simulink model "systemIndentificationLinearR2019a"  (R2019a)
settings: Solver=FixedStepAuto  StartTime=0.0  StopTime=20  RelTol=1e-3  EnableMultiTasking=on
undefined symbols (not defined in the file): sigbuilder_block
libraries: arduinolib x7, simulink x1
settings Model: SimulationMode=external  ExtModeTrigDuration=2  Creator=Win7  LastModifiedBy=manh
settings DataIOCC: SaveFormat=Array  SaveOutput=off  SaveTime=off  ReturnWorkspaceOutputs=off
settings OptimizationCC: PassReuseOutputArgsAs=Individual arguments  MaxStackSize=64
settings DebuggingCC: ParameterTunabilityLossMsg=error  ArithmeticOperatorsInVariantConditions=warning
settings HardwareCC: ProdBitPerInt=16  ProdBitPerPointer=16  ProdBitPerSizeT=16  ProdBitPerPtrDiffT=16  ProdLargestAtomicFloat=None  ProdWordSize=8  ProdHWDeviceType=Atmel->AVR
settings SFSimCC: SimUseLocalCustomCode=off  MATLABDynamicMemAlloc=off
settings RTWCC: SystemTargetFile=ert.tlc  HardwareBoard=Arduino Mega 2560  TLCOptions=-aInlineSetEventsForThisBaseRateFcn=TLC_FALSE -aSuppressMultiTaskScheduler=TLC_FALSE -aRateBasedStepFcn=1  TemplateMakefile=ert_default_tmf  GenerateReport=on  RTWUseLocalCustomCode=off  Toolchain=Arduino AVR  BuildConfiguration=Faster Runs  IncludeHyperlinkInReport=on  LaunchReport=on  GenerateTraceInfo=on  GenerateTraceReport=on  GenerateTraceReportSl=on  GenerateTraceReportSf=on  GenerateTraceReportEml=on
settings CodeAppCC: ForceParamTrailComments=on  IgnoreCustomStorageClasses=off  OperatorAnnotations=on  SimulinkDataObjDesc=on  SFDataObjDesc=on  InsertBlockDesc=on
settings ERTTargetCC: SupportContinuousTime=on  SupportVariableSizeSignals=on

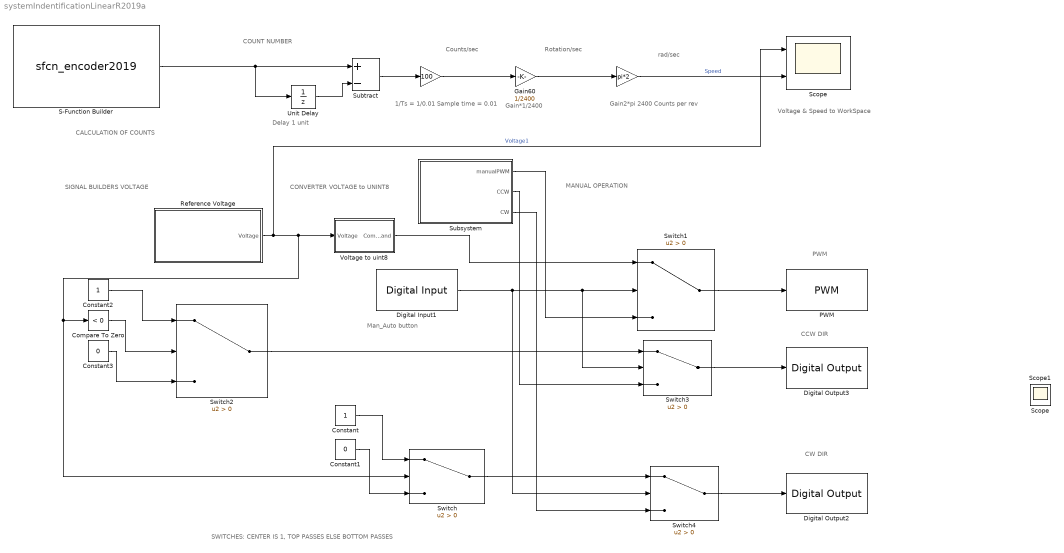
== system systemIndentificationLinearR2019a ==
  note: SIGNAL BUILDERS
      | VOLTAGE
  note: CALCULATION OF COUNTS
  note: SWITCHES: CENTER IS 1, TOP PASSES ELSE BOTTOM PASSES
  note: CONVERTER
      | VOLTAGE to UNINT8
  note: MANUAL OPERATION
  note: Voltage & Speed
      | to WorkSpace
  note: Gain2*pi
      | 2400 Counts per rev
  note: 1/Ts = 1/0.01
      | Sample time = 0.01
  note: Counts/sec
  note: Delay 1 unit
  note: CW DIR
  note: CCW DIR
  note: PWM
  note: Man_Auto button
  note: Rotation/sec
  note: rad/sec
  note: Gain*1/2400
  note: COUNT NUMBER
  " " : Gain  Gain=100  OutDataTypeStr=double
  " " : Gain  Gain=pi*2  OutDataTypeStr=double
  Compare To Zero : simulink/Logic and Bit Operations/Compare To Zero  relop=<  OutDataTypeStr=boolean
  Constant : Constant
  Constant1 : Constant  Value=0
  Constant2 : Constant
  Constant3 : Constant  Value=0
  Digital Input1 : arduinolib/Digital Input  pinNumber=28  sampleTime=0.01  blockPlatform=arduino
      settings: SourceProductName=Simulink Support Package for Arduino Hardware
  Digital Output2 : arduinolib/Digital Output  pinNumber=36  blockPlatform=arduino
  Digital Output3 : arduinolib/Digital Output  pinNumber=38  blockPlatform=arduino
  Gain60 : Gain  Gain=1/2400  OutDataTypeStr=double
  PWM : arduinolib/PWM  pinNumber=7  EnableInputFrequency=off  InitialFrequency=2000  InitialDutyCycle=0  NotificationType=None  blockPlatform=arduino
  Reference Voltage : Subsystem  Tag=STV Subsys  LoadFcn=sigbuilder_block('load');  StartFcn=sigbuilder_block('start');  StopFcn=sigbuilder_block('stop');  ClipboardFcn=sigbuilder_block('clipboard');  mask(Sigbuilder block){tuvar=[0:10]}
      mask help: Sigbuilder GUI
      mask init:
      | if ~strcmp(get_param(bdroot(gcbh),'SimulationStatus'),'stopped') tuvar = sigbuilder_block('maskInit'); end
      settings: CopyFcn=sigbuilder_block('copy');  DeleteFcn=sigbuilder_block('delete');  ModelCloseFcn=sigbuilder_block('modelClose');  PreSaveFcn=sigbuilder_block('preSave');  PauseFcn=sigbuilder_block('pause')  ContinueFcn=sigbuilder_block('continue')  NameChangeFcn=sigbuilder_block('namechange');  OpenFcn=sigbuilder_block('open',[105 207 438 216 ]);  CloseFcn=sigbuilder_block('close');
      mask Display: plot(0, 0, 100, 100,[2, 2, 32, 32, 2], [68, 8, 8, 68, 68],[32, 2], [38, 38], [32, 19, 2],[53, 60, 44], [32, 17, 17, 2],[16, 16, 31, 31]);txt = getActiveGroup(gcbh);text(2, 100, txt,'verticalAlignment', 'top');
  S-Function Builder : S-Function  FunctionName=sfcn_encoder2019  Parameters=uint8(0),uint8(2),uint8(3)  SFunctionModules=sfcn_encoder2019_wrapper  SFunctionDeploymentMode=off  EnableBusSupport=off  mask(S-Function Builder){}
      mask help: Simulink:masks:SFunctionBuilder_MD
      mask init:
      | val = [[.9  0.75 0.75 1 1 .9 .9 1]',[1 1 0.75 0.75 .9 .9 1 .9]'];try , sys = get_param(gcb,'SfunBuilderFcnName');if isempty(sys), sys = get_param(gcb,'FunctionName'); end,catch, sys = get_param(gcb,'FunctionName'); end
      settings: CopyFcn=set_param(gcbh,'LinkStatus','none')  PreSaveFcn=try, set_param(gcb,'FunctionName','sfcn_encoder2019'), end  OpenFcn=sfunctionwizard(gcbh)
      mask Display: plot(val(:,1),val(:,2)),disp(sys), port_label('output',1,'pos')
  "Scope " : Scope  NumInputPorts=2
  Subsystem : Subsystem
  Subtract : Sum  Inputs=+-
  Switch{,1..4} (5 alike) : Switch  Criteria=u2 > Threshold
  Unit Delay : UnitDelay  SampleTime=-1  HasFrameUpgradeWarning=on
  Voltage to uint8 : Subsystem
  Scope : Scope
  Scope1 : Scope
  wires:
  Reference Voltage/1(Voltage) -> "Scope "/1, Switch/2, Compare To Zero/1, Voltage to uint8/1(Voltage)  "Voltage1"
  Compare To Zero/1 -> Switch2/2
  Constant/1 -> Switch/1
  Constant1/1 -> Switch/3
  Constant2/1 -> Switch2/1
  Constant3/1 -> Switch2/3
  Digital Input1/1 -> Switch1/2, Switch3/2, Switch4/2
  Voltage to uint8/1(Command) -> Switch1/1
  Switch2/1 -> Switch3/1
  Switch/1 -> Switch4/1
  Subsystem/1(manualPWM) -> Switch1/3
  Subsystem/2(CCW) -> Switch3/3
  Subsystem/3(CW) -> Switch4/3
  Switch3/1 -> Digital Output3/1
  Switch4/1 -> Digital Output2/1
  Switch1/1 -> PWM/1
  S-Function Builder/1 -> Subtract/1, Unit Delay/1
  Unit Delay/1 -> Subtract/2
  Gain60/1 -> " "/1
  " "/1 -> "Scope "/2  "Speed"
  Subtract/1 -> " "/1
  " "/1 -> Gain60/1

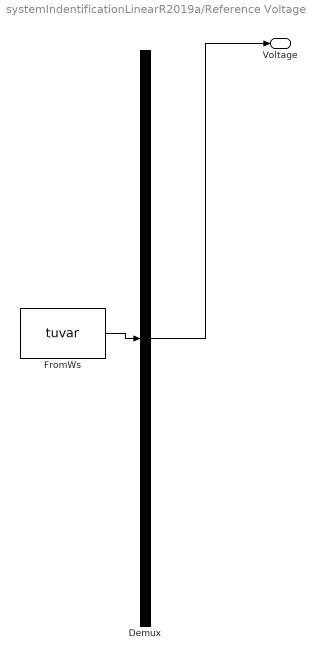
== system systemIndentificationLinearR2019a/Reference Voltage ==
  Demux : Demux  Tag=STV Demux  Outputs=1
  FromWs : FromWorkspace  Tag=STV FromWs  VariableName=tuvar  SampleTime=1/100  OutputAfterFinalValue=Setting to zero
      SigBuilderData=|
      | common.afterFinalStr = 'Set to zero'
      | common.sampleTime = '1/100'
      | dataSet(1).timeRange = [0 20]
      | dataSet(1).name = 'Bounds12'
      | dataSet(2).timeRange = [0 10]
      | dataSet(2).name = 'Bounds1'
      | dataSet(3).timeRange = [0 20]
      | dataSet(3).name = 'Sine3'
      | dataSet(4).timeRange = [0 20]
      | dataSet(4).name = 'Sine5'
      | dataSet(5).timeRange = [0 20]
      | dataSet(5).name = 'Step1'
      | dataSet(6).timeRange = [0 20]
      | dataSet(6).name = 'Step2'
      | dataSet(7).timeRange = [0 10]
      | dataSet(7).name = 'RampSquare'
      | dataSet(8).timeRange = [0 10]
      | dataSet(8).name = 'Steps'
      | dataSet(9).timeRange = [0 10]
      | dataSet(9).name = 'Small Steps'
      | dataSet(10).timeRange = [0 10]
      | dataSet(10).name = 'Square'
      | dataSet(11).timeRange = [0 55]
      | dataSet(11).name = 'DeadZone'
      | sbobj.Groups(1).Name = 'Bounds12'
      | sbobj.Groups(1).Signals.Name = 'Voltage'
      | sbobj.Groups(1).Signals.XData = [0 2 2 9 9 11 11 18 18 20]
      | sbobj.Groups(1).Signals.YData = [0 0 12 12 0 0 -12 -12 0 0]
      | sbobj.Groups(1).TimeRange = [0 20]
      | sbobj.Groups(2).Name = 'Bounds1'
      | sbobj.Groups(2).Signals.Name = 'Voltage'
      | sbobj.Groups(2).Signals.XData = [0 2.5 2.5 5 5 7.5 7.5 10]
      | sbobj.Groups(2).Signals.YData = [1 1 -1 -1 1 1 -1 -1]
      | sbobj.Groups(3).Name = 'Sine3'
      | sbobj.Groups(3).Signals.Name = 'Voltage'
      | sbobj.Groups(3).Signals.XData = [0 0.01 0.02 0.03 0.04 0.05 0.06 0.07 0.08 0.09 0.1 0.11 ... (2001 elements, 1x2001)]
      | sbobj.Groups(3).Signals.YData = [0 0.0299995000025 0.05999600008 0.0899865006075 0.11996800256 0.149937507812 0.179892019438 0.209828542013 0.239744081908 0.269635647594 0.29950024994 0.329334902512 ... (2001 elements, 1x2001)]
      | sbobj.Groups(3).TimeRange = [0 20]
      | sbobj.Groups(4).Name = 'Sine5'
      | sbobj.Groups(4).Signals.Name = 'Voltage'
      | sbobj.Groups(4).Signals.XData = [0 0.01 0.02 0.03 0.04 0.05 0.06 0.07 0.08 0.09 0.1 0.11 ... (2001 elements, 1x2001)]
      | sbobj.Groups(4).Signals.YData = [0 0.0499991666708 0.0999933334667 0.149977501012 0.199946670933 0.249895846353 0.299820032397 0.349714236688 0.399573469846 0.44939274599 0.499167083234 0.548891504186 ... (2001 elements, 1x2001)]
      | sbobj.Groups(4).TimeRange = [0 20]
      | sbobj.Groups(5).Name = 'Step1'
      | sbobj.Groups(5).Signals.Name = 'Voltage'
      | sbobj.Groups(5).Signals.XData = [0 0.01 0.02 0.03 0.04 0.05 0.06 0.07 0.08 0.09 0.1 0.11 ... (2001 elements, 1x2001)]
      | sbobj.Groups(5).Signals.YData = [0 0 0 0 0 0 0 0 0 0 0 0 ... (2001 elements, 1x2001)]
      | sbobj.Groups(5).TimeRange = [0 20]
      | sbobj.Groups(6).Name = 'Step2'
      | sbobj.Groups(6).Signals.Name = 'Voltage'
      | sbobj.Groups(6).Signals.XData = [0 0.01 0.02 0.03 0.04 0.05 0.06 0.07 0.08 0.09 0.1 0.11 ... (2001 elements, 1x2001)]
      | sbobj.Groups(6).Signals.YData = [0 0 0 0 0 0 0 0 0 0 0 0 ... (2001 elements, 1x2001)]
      | sbobj.Groups(6).TimeRange = [0 20]
      | sbobj.Groups(7).Name = 'RampSquare'
      | sbobj.Groups(7).Signals.Name = 'Voltage'
      | sbobj.Groups(7).Signals.XData = [0 1 1 2 2 3 3 4 4 5 5 6 6 7 7 8 8 9 9 9.8 9.8 10]
      | sbobj.Groups(7).Signals.YData = [0 0.75 0 -0.75 0 1.5 0 -1.5 2 2 -2 -2 3 3 -3 -3 1 1 -1 -1 0 0]
      | sbobj.Groups(8).Name = 'Steps'
      | sbobj.Groups(8).Signals.Name = 'Voltage'
      | sbobj.Groups(8).Signals.XData = [0 1.52 1.52 2.4 2.4 3.66 3.68 4.64 4.64 6.02 6.02 7 7 8.96 8.96 10]
      | sbobj.Groups(8).Signals.YData = [2 2 -3 -3 3 -1 1.95 1.95 -2 -2 0.7 0.7 -1.05 -0.05 0 0]
      | sbobj.Groups(9).Name = 'Small Steps'
      | sbobj.Groups(9).Signals.Name = 'Voltage'
      | sbobj.Groups(9).Signals.XData = [0 0.5 0.5 1.02 1.02 2 2 2.58 2.58 3.78 3.78 4.64 4.64 5.28 5.28 6 6 7 7 9 9 10]
      | sbobj.Groups(9).Signals.YData = [0.4 0.4 0.75 0.75 1.5 3 1.55 1.55 3.55 3.55 -3.05 -3.05 -1 -1 -0.45 -0.45 0.7 0.7 -2.05 -0.05 1 1]
      | sbobj.Groups(10).Name = 'Square'
      | sbobj.Groups(10).Signals.Name = 'Voltage'
      | sbobj.Groups(10).Signals.XData = [0 0.5 0.5 1.02 1.02 1.5 1.5 2 2 2.5 2.5 3 3 4 4 5 5 6 6 7 7 8 8 9 9 9.8 9.8 10]
      | sbobj.Groups(10).Signals.YData = [0.4 0.4 -0.4 -0.4 1 1 -1 -1 1.5 1.5 -1.5 -1.5 2 2 -2 -2 3 3 -3 -3 1.3 1.3 -1.3 -1.3 -4 -4 0 0]
      | sbobj.Groups(11).Name = 'DeadZone'
      | sbobj.Groups(11).Signals.Name = 'Voltage'
      | sbobj.Groups(11).Signals.XData = [0 5 5 10 10 15 15 20 25 30 30 35 40 45 50 50 55]
      | sbobj.Groups(11).Signals.YData = [0 0 0.16 0.16 0.3 0.3 0.7 0.7 -0.205 -0.205 -0.355 -0.35 -0.605 -0.605 0.005 0 0]
      | sbobj.Groups(11).TimeRange = [0 55]
  Voltage : Outport  Tag=STV Outport
  wires:
  Demux/1 -> Voltage/1
  FromWs/1 -> Demux/1

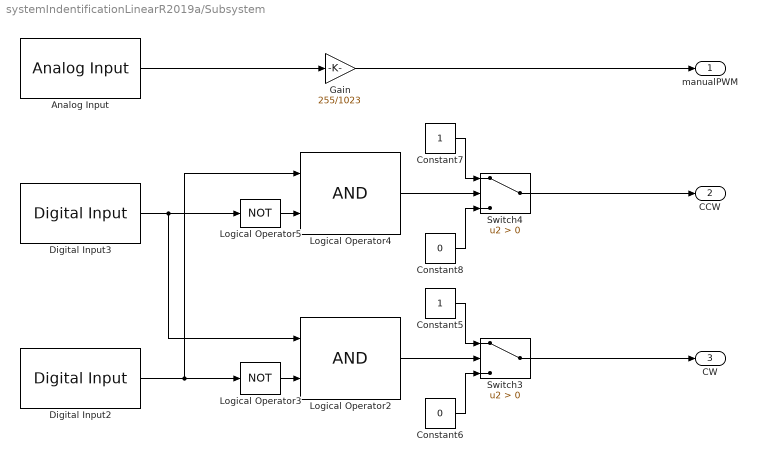
== system systemIndentificationLinearR2019a/Subsystem ==
  Analog Input : arduinolib/Analog Input  pinNumber=5  ReadResultsOnly=off  ConversionTriggerSource=Software  ExternalTriggerType=uint32(0)  OutputDataType=uint16  EnableConversionCompleteNotify=off  EnableOuputStatus=off  SampleTime=0.01  blockPlatform=arduino
  Constant5 : Constant
  Constant6 : Constant  Value=0
  Constant7 : Constant
  Constant8 : Constant  Value=0
  Digital Input2 : arduinolib/Digital Input  pinNumber=22  sampleTime=0.01  blockPlatform=arduino
      settings: SourceProductName=Simulink Support Package for Arduino Hardware
  Digital Input3 : arduinolib/Digital Input  pinNumber=24  sampleTime=0.01  blockPlatform=arduino
      settings: SourceProductName=Simulink Support Package for Arduino Hardware
  Gain : Gain  Gain=255/1023
  Logical Operator2 : Logic  AllPortsSameDT=off  OutDataTypeStr=boolean
  Logical Operator3 : Logic  Operator=NOT  AllPortsSameDT=off  OutDataTypeStr=boolean
  Logical Operator4 : Logic  AllPortsSameDT=off  OutDataTypeStr=boolean
  Logical Operator5 : Logic  Operator=NOT  AllPortsSameDT=off  OutDataTypeStr=boolean
  Switch3 : Switch  Criteria=u2 > Threshold
  Switch4 : Switch  Criteria=u2 > Threshold
  manualPWM : Outport
  CCW : Outport  Port=2
  CW : Outport  Port=3
  wires:
  Constant6/1 -> Switch3/3
  Constant7/1 -> Switch4/1
  Logical Operator5/1 -> Logical Operator4/2
  Constant5/1 -> Switch3/1
  Switch3/1 -> CW/1
  Logical Operator3/1 -> Logical Operator2/2
  Logical Operator2/1 -> Switch3/2
  Switch4/1 -> CCW/1
  Digital Input2/1 -> Logical Operator4/1, Logical Operator3/1
  Gain/1 -> manualPWM/1
  Analog Input/1 -> Gain/1
  Logical Operator4/1 -> Switch4/2
  Digital Input3/1 -> Logical Operator5/1, Logical Operator2/1
  Constant8/1 -> Switch4/3

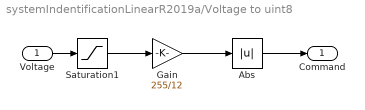
== system systemIndentificationLinearR2019a/Voltage to uint8 ==
  Voltage : Inport
  Abs : Abs  OutDataTypeStr=uint8
  Gain : Gain  Gain=255/12  OutDataTypeStr=single
  Saturation1 : Saturate  UpperLimit=12  LowerLimit=-12
  Command : Outport
  wires:
  Voltage/1 -> Saturation1/1
  Saturation1/1 -> Gain/1
  Gain/1 -> Abs/1
  Abs/1 -> Command/1
